simulink model "Simple_bjt"  (R2018b)
settings: Solver=FixedStepDiscrete  StartTime=0.0  StopTime=10  FixedStep=Ts  RelTol=1e-3
PreLoadFcn:
  | Ts = 1e-3
undefined symbols (not defined in the file or in its folder): DiscIntNeverNeededParam, sigbuilder_block
libraries: Simple_lib x13
settings Model: PauseTimes=455  Creator=billw  LastModifiedBy=billw
settings DataIOCC: SaveOutput=off  DSMLogging=off  SaveTime=off

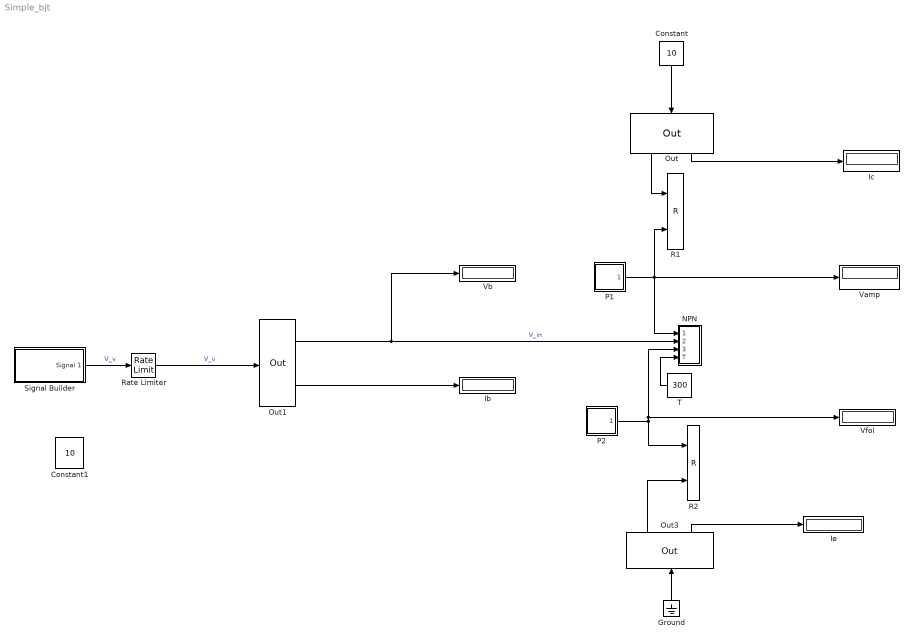
== system Simple_bjt ==
  Constant : Constant  Value=10
  Constant1 : Constant  Value=10
  Ground : Ground
  Ib : Display
  Ic : Display
  Ie : Display
  NPN : Subsystem  AncestorBlock=Simple_lib/Electronics/NPN  mask{alpha_F=0.98, alpha_R=0.9}
      mask Display:
      | patch([0 0 0.1 0.1],[-.7 1 1 -.7])
      | patch([0 0 0.1 0.1],[-1 -.7 -.7 -1],[.9 .5 .1])
      | 
      | plot([0 1],[0.25 1])
      | plot([0 1],[-0.25 -1])
      | 
      | patch([.8 1 1],[-1 -1 -0.8])
  Out : Simple_lib/Electronics/Out  Tag=Electrical
      mask init:
      | initOutput
      mask Display:
      | % This is a new mask on top of the base mask.
      | % Use "View base mask" link below to see the base mask.
      | % Icon for flow out
      | %% Complex icon
      | %plot([0 1 1], [0 0 0.4])
      | %plot([1 1 3], [0.6 1 1])
      | %plot([1 3 2 1 0 2], [0.6 0.6 0.4 0.6 0.4 0.4])
      | %patch([0 2 1],[0.4 0.4 0.6])
      | %plot([3 2 2], [1 1 0.6])
      | %plot([2.2 2.2], [1 0.6])
      | %plot([1.8 1.8], [1 0.6])
      | %plot([1.6 2.4], [0 0])
      | %plot([2 2], [0.1 -0.1])
      | %plot([2 2], [0.4 0.2])
      | %plot([2 2 3], [-0.2 -1 -1])
      | 
      | %color('white')
      | %plot([0 3], [2 2])
      | %plot([0 3], [-2 -2])
      | 
      | %% Bolder icon
      | plot([-1 0 1], [0 -1 0])
      | %patch([-1 1 0 -1], [1 1 2 1]*1-1)
      | patch([-1 -.2 -.2], [0 0 1])
      | patch([1 .2 .2], [0 0 1])
      | %patch( [-0.1 0.1 0.1 -0.1], [0 0 1 1], [1 1 1])
      | 
      | color('white')
      | plot( [-1 1], [2 2])
      | plot( [-1 1], -[2 2])
  Out1 : Simple_lib/Electronics/Out  Tag=Electrical
      mask init:
      | initOutput
      mask Display:
      | % This is a new mask on top of the base mask.
      | % Use "View base mask" link below to see the base mask.
      | % Icon for flow out
      | %% Complex icon
      | %plot([0 1 1], [0 0 0.4])
      | %plot([1 1 3], [0.6 1 1])
      | %plot([1 3 2 1 0 2], [0.6 0.6 0.4 0.6 0.4 0.4])
      | %patch([0 2 1],[0.4 0.4 0.6])
      | %plot([3 2 2], [1 1 0.6])
      | %plot([2.2 2.2], [1 0.6])
      | %plot([1.8 1.8], [1 0.6])
      | %plot([1.6 2.4], [0 0])
      | %plot([2 2], [0.1 -0.1])
      | %plot([2 2], [0.4 0.2])
      | %plot([2 2 3], [-0.2 -1 -1])
      | 
      | %color('white')
      | %plot([0 3], [2 2])
      | %plot([0 3], [-2 -2])
      | 
      | %% Bolder icon
      | plot([-1 0 1], [0 -1 0])
      | %patch([-1 1 0 -1], [1 1 2 1]*1-1)
      | patch([-1 -.2 -.2], [0 0 1])
      | patch([1 .2 .2], [0 0 1])
      | %patch( [-0.1 0.1 0.1 -0.1], [0 0 1 1], [1 1 1])
      | 
      | color('white')
      | plot( [-1 1], [2 2])
      | plot( [-1 1], -[2 2])
  Out3 : Simple_lib/Electronics/Out  Tag=Electrical
      mask init:
      | initOutput
      mask Display:
      | % This is a new mask on top of the base mask.
      | % Use "View base mask" link below to see the base mask.
      | % Icon for flow out
      | %% Complex icon
      | %plot([0 1 1], [0 0 0.4])
      | %plot([1 1 3], [0.6 1 1])
      | %plot([1 3 2 1 0 2], [0.6 0.6 0.4 0.6 0.4 0.4])
      | %patch([0 2 1],[0.4 0.4 0.6])
      | %plot([3 2 2], [1 1 0.6])
      | %plot([2.2 2.2], [1 0.6])
      | %plot([1.8 1.8], [1 0.6])
      | %plot([1.6 2.4], [0 0])
      | %plot([2 2], [0.1 -0.1])
      | %plot([2 2], [0.4 0.2])
      | %plot([2 2 3], [-0.2 -1 -1])
      | 
      | %color('white')
      | %plot([0 3], [2 2])
      | %plot([0 3], [-2 -2])
      | 
      | %% Bolder icon
      | plot([-1 0 1], [0 -1 0])
      | %patch([-1 1 0 -1], [1 1 2 1]*1-1)
      | patch([-1 -.2 -.2], [0 0 1])
      | patch([1 .2 .2], [0 0 1])
      | %patch( [-0.1 0.1 0.1 -0.1], [0 0 1 1], [1 1 1])
      | 
      | color('white')
      | plot( [-1 1], [2 2])
      | plot( [-1 1], -[2 2])
  P1 : Subsystem  AncestorBlock=Simple_lib/Electronics/P
      mask Display: disp(get(gcbh,'Name'))
  P2 : Subsystem  AncestorBlock=Simple_lib/Electronics/P
      mask Display: disp(get(gcbh,'Name'))
  R1 : Simple_lib/Electronics/R  R=5e3
      settings: AttributesFormatString=%<R> Ohms
  R2 : Simple_lib/Electronics/R  R=1e3
      settings: AttributesFormatString=%<R> Ohms
  Rate Limiter : RateLimiter  RisingSlewLimit=10  FallingSlewLimit=-10  SampleTimeMode=inherited  LinearizeAsGain=off
  Signal Builder : Subsystem  Tag=STV Subsys  LoadFcn=sigbuilder_block('load',[342 162.6 550.8 400.2 ]);  StartFcn=sigbuilder_block('start');  StopFcn=sigbuilder_block('stop');  ClipboardFcn=sigbuilder_block('clipboard');  mask(Sigbuilder block){tuvar=[0:10]}
      mask help: Simulink:masks:SigbuilderBlock_MD
      mask init:
      | if ~strcmp(get_param(bdroot(gcbh),'SimulationStatus'),'stopped') tuvar = sigbuilder_block('maskInit'); end
      settings: CopyFcn=sigbuilder_block('copy');  DeleteFcn=sigbuilder_block('delete');  ModelCloseFcn=sigbuilder_block('modelClose');  PreSaveFcn=sigbuilder_block('preSave');  PauseFcn=sigbuilder_block('pause');  ContinueFcn=sigbuilder_block('continue');  NameChangeFcn=sigbuilder_block('namechange');  OpenFcn=sigbuilder_block('open',[437.6 199.2 550.4 400 ]);  CloseFcn=sigbuilder_block('close');
      mask Display: plot(0, 0, 100, 100,[2, 2, 32, 32, 2], [68, 8, 8, 68, 68],[32, 2], [38, 38], [32, 19, 2],[53, 60, 44], [32, 17, 17, 2],[16, 16, 31, 31]);txt = getActiveGroup(gcbh);text(2, 100, txt,'verticalAlignment', 'top');
  T : Constant  Value=300
  Vamp : Display
  Vb : Display
  Vfol : Display
  wires:
  Signal Builder/1(Signal 1) -> Rate Limiter/1  "V_v"
  P1/1(Out1) -> R1/2, Vamp/1, NPN/1(Collector)
  Out/2 -> Ic/1
  Out3/1 -> R2/2
  Out1/1 -> Vb/1, NPN/2(Base)  "V_in"
  Constant/1 -> Out/1
  Out1/2 -> Ib/1
  Out/1 -> R1/1
  T/1 -> NPN/4(T)
  P2/1(Out1) -> NPN/3(Emitter), Vfol/1, R2/1
  Rate Limiter/1 -> Out1/1  "V_v"
  Ground/1 -> Out3/1
  Out3/2 -> Ie/1

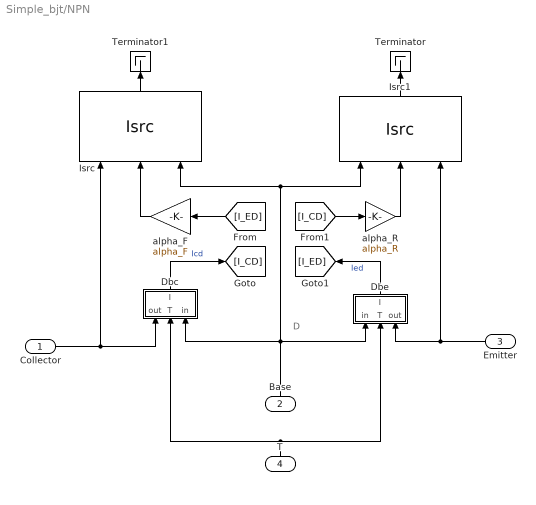
== system Simple_bjt/NPN ==
  note: D
  Collector : Inport
  Base : Inport  Port=2
  Emitter : Inport  Port=3
  T : Inport  Port=4
  Dbc : Subsystem  AncestorBlock=Simple_lib/Electronics/D  mask{I_S=1e-12}
      mask Display:
      | %plot( [ -1 0 0 ],[-1 -1 -0.3 ])
      | %plot( [ 0 0 -1],[ 0.3 1 1])
      | plot( [ -1 1],-[1 1]*1.3)
      | plot([-1 1 0 -1],[1 1 -1 1]*1.3)
      | color('white')
      | plot([-1 1], [-2 -2])
      | plot([-1 1], [2 2])
      | %port_label('input', 1, '1')
  Dbe : Subsystem  AncestorBlock=Simple_lib/Electronics/D  mask{I_S=1e-12}
      mask Display:
      | %plot( [ -1 0 0 ],[-1 -1 -0.3 ])
      | %plot( [ 0 0 -1],[ 0.3 1 1])
      | plot( [ -1 1],-[1 1]*1.3)
      | plot([-1 1 0 -1],[1 1 -1 1]*1.3)
      | color('white')
      | plot([-1 1], [-2 -2])
      | plot([-1 1], [2 2])
      | %port_label('input', 1, '1')
  Isrc : Simple_lib/Electronics/Isrc  SystemSampleTime=-1
  Isrc1 : Simple_lib/Electronics/Isrc  SystemSampleTime=-1
  Terminator : Terminator
  Terminator1 : Terminator
  alpha_F : Gain  Gain=alpha_F
  alpha_R : Gain  Gain=alpha_R
  wires:
  T/1 -> Dbc/2(T), Dbe/2(T)
  Base/1 -> Dbe/1(in), Isrc1/3, Isrc/3, Dbc/1(in)
  Dbe/1(I) -> [I_ED]  "Ied"
  alpha_R/1 -> Isrc1/2
  [I_CD] -> alpha_R/1
  alpha_F/1 -> Isrc/2
  [I_ED] -> alpha_F/1
  Dbc/1(I) -> [I_CD]  "Icd"
  Collector/1 -> Isrc/1, Dbc/3(out)
  Emitter/1 -> Dbe/3(out), Isrc1/1
  Isrc1/1 -> Terminator/1
  Isrc/1 -> Terminator1/1

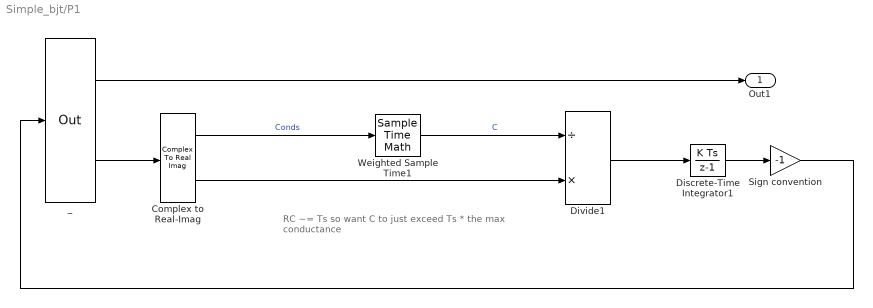
== system Simple_bjt/P1 ==
  note: RC ~= Ts
      | so want C to just exceed Ts * the max conductance
  Complex to Real-Imag : ComplexToRealImag
  Discrete-Time Integrator1 : DiscreteIntegrator  gainval=1  SampleTime=-1  LimitOutput=on  UpperSaturationLimit=1e3  LowerSaturationLimit=-1e3  ICPrevOutput=DiscIntNeverNeededParam  ICPrevScaledInput=DiscIntNeverNeededParam
  Divide1 : Product  Inputs=/*
  Sign convention : Gain  Gain=-1
  Weighted Sample Time1 : SampleTimeMath  TsampMathOp=*  weightValue=uu
  _ : Simple_lib/Electronics/Out  Tag=Electrical
      mask init:
      | initOutput
      mask Display:
      | % This is a new mask on top of the base mask.
      | % Use "View base mask" link below to see the base mask.
      | % Icon for flow out
      | %% Complex icon
      | %plot([0 1 1], [0 0 0.4])
      | %plot([1 1 3], [0.6 1 1])
      | %plot([1 3 2 1 0 2], [0.6 0.6 0.4 0.6 0.4 0.4])
      | %patch([0 2 1],[0.4 0.4 0.6])
      | %plot([3 2 2], [1 1 0.6])
      | %plot([2.2 2.2], [1 0.6])
      | %plot([1.8 1.8], [1 0.6])
      | %plot([1.6 2.4], [0 0])
      | %plot([2 2], [0.1 -0.1])
      | %plot([2 2], [0.4 0.2])
      | %plot([2 2 3], [-0.2 -1 -1])
      | 
      | %color('white')
      | %plot([0 3], [2 2])
      | %plot([0 3], [-2 -2])
      | 
      | %% Bolder icon
      | plot([-1 0 1], [0 -1 0])
      | %patch([-1 1 0 -1], [1 1 2 1]*1-1)
      | patch([-1 -.2 -.2], [0 0 1])
      | patch([1 .2 .2], [0 0 1])
      | %patch( [-0.1 0.1 0.1 -0.1], [0 0 1 1], [1 1 1])
      | 
      | color('white')
      | plot( [-1 1], [2 2])
      | plot( [-1 1], -[2 2])
  Out1 : Outport
  wires:
  Sign convention/1 -> _/1
  Complex to Real-Imag/2 -> Divide1/2
  Complex to Real-Imag/1 -> Weighted Sample Time1/1  "Conds"
  Divide1/1 -> Discrete-Time Integrator1/1
  Discrete-Time Integrator1/1 -> Sign convention/1
  _/2 -> Complex to Real-Imag/1
  _/1 -> Out1/1
  Weighted Sample Time1/1 -> Divide1/1  "C"

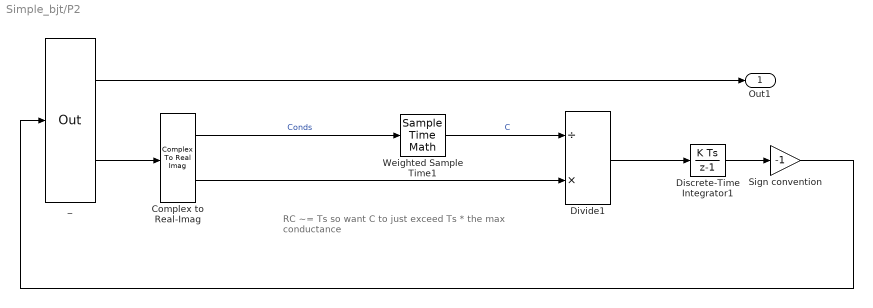
== system Simple_bjt/P2 ==
  note: RC ~= Ts
      | so want C to just exceed Ts * the max conductance
  Complex to Real-Imag : ComplexToRealImag
  Discrete-Time Integrator1 : DiscreteIntegrator  gainval=1  SampleTime=-1  LimitOutput=on  UpperSaturationLimit=1e3  LowerSaturationLimit=-1e3  ICPrevOutput=DiscIntNeverNeededParam  ICPrevScaledInput=DiscIntNeverNeededParam
  Divide1 : Product  Inputs=/*
  Sign convention : Gain  Gain=-1
  Weighted Sample Time1 : SampleTimeMath  TsampMathOp=*  weightValue=uu
  _ : Simple_lib/Electronics/Out  Tag=Electrical
      mask init:
      | initOutput
      mask Display:
      | % This is a new mask on top of the base mask.
      | % Use "View base mask" link below to see the base mask.
      | % Icon for flow out
      | %% Complex icon
      | %plot([0 1 1], [0 0 0.4])
      | %plot([1 1 3], [0.6 1 1])
      | %plot([1 3 2 1 0 2], [0.6 0.6 0.4 0.6 0.4 0.4])
      | %patch([0 2 1],[0.4 0.4 0.6])
      | %plot([3 2 2], [1 1 0.6])
      | %plot([2.2 2.2], [1 0.6])
      | %plot([1.8 1.8], [1 0.6])
      | %plot([1.6 2.4], [0 0])
      | %plot([2 2], [0.1 -0.1])
      | %plot([2 2], [0.4 0.2])
      | %plot([2 2 3], [-0.2 -1 -1])
      | 
      | %color('white')
      | %plot([0 3], [2 2])
      | %plot([0 3], [-2 -2])
      | 
      | %% Bolder icon
      | plot([-1 0 1], [0 -1 0])
      | %patch([-1 1 0 -1], [1 1 2 1]*1-1)
      | patch([-1 -.2 -.2], [0 0 1])
      | patch([1 .2 .2], [0 0 1])
      | %patch( [-0.1 0.1 0.1 -0.1], [0 0 1 1], [1 1 1])
      | 
      | color('white')
      | plot( [-1 1], [2 2])
      | plot( [-1 1], -[2 2])
  Out1 : Outport
  wires:
  Sign convention/1 -> _/1
  Complex to Real-Imag/2 -> Divide1/2
  Complex to Real-Imag/1 -> Weighted Sample Time1/1  "Conds"
  Divide1/1 -> Discrete-Time Integrator1/1
  Discrete-Time Integrator1/1 -> Sign convention/1
  _/2 -> Complex to Real-Imag/1
  _/1 -> Out1/1
  Weighted Sample Time1/1 -> Divide1/1  "C"

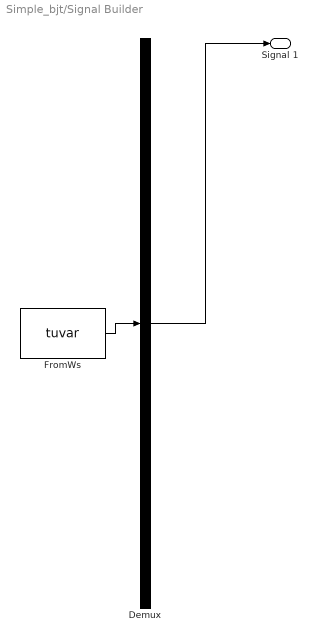
== system Simple_bjt/Signal Builder ==
  Demux : Demux  Tag=STV Demux  Outputs=1
  FromWs : FromWorkspace  Tag=STV FromWs  VariableName=tuvar  SampleTime=0
      SigBuilderData=|
      | common.afterFinalStr = 'Extrapolate'
      | common.sampleTime = 0
      | dataSet.timeRange = [0 10]
      | dataSet.name = 'Group 1'
      | sbobj.Groups.Name = 'Group 1'
      | sbobj.Groups.Signals.Name = 'Signal 1'
      | sbobj.Groups.Signals.XData = [0 0.96 0.96 2 2 4 4 6 6 7 7 7.98 7.98 10]
      | sbobj.Groups.Signals.YData = [0 0 0.3 0.3 0 0 0.395 1.44 0 0 8.75 8.75 0 0]
  Signal 1 : Outport  Tag=STV Outport
  wires:
  Demux/1 -> Signal 1/1
  FromWs/1 -> Demux/1

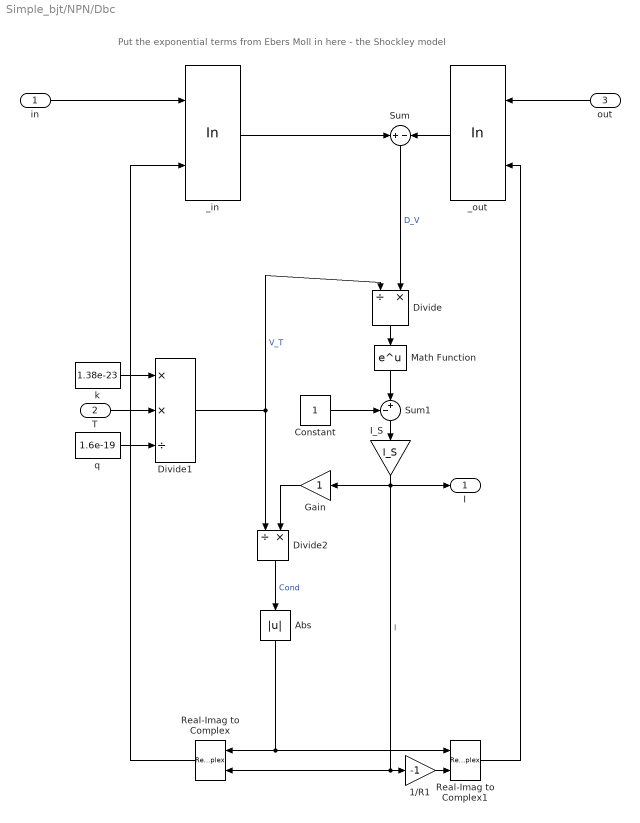
== system Simple_bjt/NPN/Dbc ==
  note: Put the exponential terms from Ebers Moll in here - the Shockley model
  in : Inport
  T : Inport  Port=2
  out : Inport  Port=3
  1/R1 : Gain  Gain=-1
  Abs : Abs
  Constant : Constant
  Divide : Product  Inputs=/*
  Divide1 : Product  Inputs=**/
  Divide2 : Product  Inputs=/*
  Gain : Gain
  I_S : Gain  Gain=I_S
  Math Function : Math  SaturateOnIntegerOverflow=on
  Real-Imag to Complex : RealImagToComplex
  Real-Imag to Complex1 : RealImagToComplex
  Sum : Sum  Inputs=+|-
  Sum1 : Sum  Inputs=-+|
  _in : Simple_lib/Electronics/In
      mask init:
      | initInput
      mask Display:
      | % This is a new mask on top of the base mask.
      | % Use "View base mask" link below to see the base mask.
      | %% Icon for flow in
      | % Signally design
      | %plot([0 2 2 3], [1 1 0 0])
      | %plot([1 3 2 1 0 2], [0.6 0.6 0.4 0.6 0.4 0.4])
      | %patch([1 3 2],[0.6 0.6 0.4])
      | %plot([0 1 1], [1 1 0.6])
      | %plot([1 1 0], [0.4 -1 -1])
      | 
      | %color('white')
      | %plot([0 3], [2 2])
      | %plot([0 3], [-2 -2])
      | 
      | %% Bolder design
      | %patch( [0 1 -1], [0 1 1])
      | patch( [-0.1 -0.1 -1], [0.95 0 0.95])
      | patch( [0.1 0.1 1], [1 0 1])
      | plot( [0.1 1 -1 -0.1], [0 -2 -2 0]*0.5)
      | %patch( [-0.1 0.1 0.1 -0.1], [0 0 1 1], [1 1 1])
      | %patch( [-1 0.1 0.1 -1], [1 1 0.95 0.95], [1 1 1])
      | 
      | %% Size the box
      | color('white')
      | plot( [-1 1], [2 2])
      | plot( [-1 1], -[2 2])
  _out : Simple_lib/Electronics/In
      mask init:
      | initInput
      mask Display:
      | % This is a new mask on top of the base mask.
      | % Use "View base mask" link below to see the base mask.
      | %% Icon for flow in
      | % Signally design
      | %plot([0 2 2 3], [1 1 0 0])
      | %plot([1 3 2 1 0 2], [0.6 0.6 0.4 0.6 0.4 0.4])
      | %patch([1 3 2],[0.6 0.6 0.4])
      | %plot([0 1 1], [1 1 0.6])
      | %plot([1 1 0], [0.4 -1 -1])
      | 
      | %color('white')
      | %plot([0 3], [2 2])
      | %plot([0 3], [-2 -2])
      | 
      | %% Bolder design
      | %patch( [0 1 -1], [0 1 1])
      | patch( [-0.1 -0.1 -1], [0.95 0 0.95])
      | patch( [0.1 0.1 1], [1 0 1])
      | plot( [0.1 1 -1 -0.1], [0 -2 -2 0]*0.5)
      | %patch( [-0.1 0.1 0.1 -0.1], [0 0 1 1], [1 1 1])
      | %patch( [-1 0.1 0.1 -1], [1 1 0.95 0.95], [1 1 1])
      | 
      | %% Size the box
      | color('white')
      | plot( [-1 1], [2 2])
      | plot( [-1 1], -[2 2])
  k : Constant  Value=1.38e-23
  q : Constant  Value=1.6e-19
  I : Outport
  wires:
  Real-Imag to Complex1/1 -> _out/2
  Divide2/1 -> Abs/1  "Cond"
  I_S/1 -> Real-Imag to Complex/2, 1/R1/1, Gain/1, I/1  "I"
  _out/1 -> Sum/2
  Math Function/1 -> Sum1/2
  Constant/1 -> Sum1/1
  Sum1/1 -> I_S/1
  out/1 -> _out/1
  Sum/1 -> Divide/2  "D_V"
  _in/1 -> Sum/1
  in/1 -> _in/1
  Divide/1 -> Math Function/1
  T/1 -> Divide1/2
  q/1 -> Divide1/3
  Divide1/1 -> Divide2/1, Divide/1  "V_T"
  k/1 -> Divide1/1
  Gain/1 -> Divide2/2
  Abs/1 -> Real-Imag to Complex1/1, Real-Imag to Complex/1
  Real-Imag to Complex/1 -> _in/2
  1/R1/1 -> Real-Imag to Complex1/2

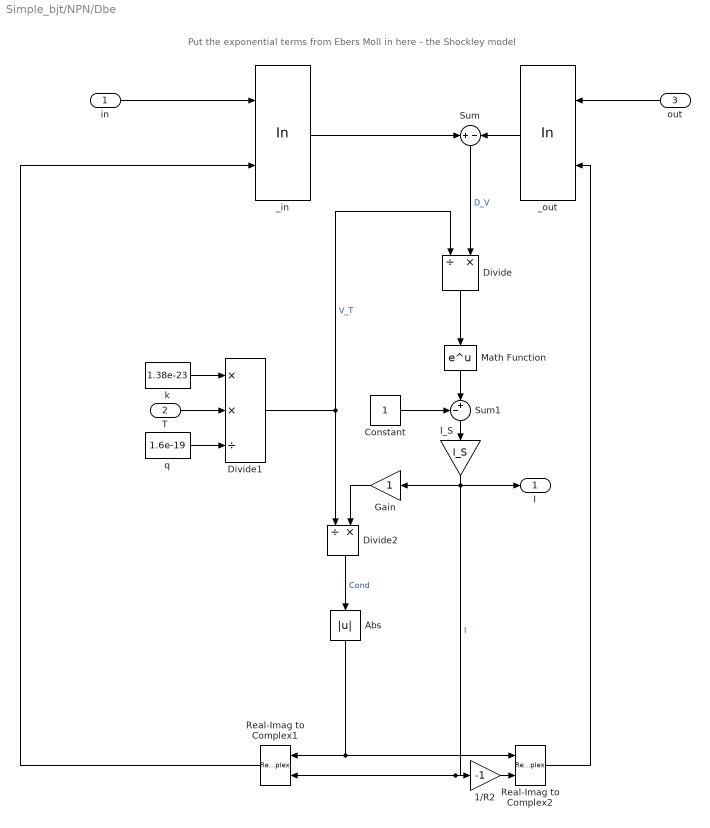
== system Simple_bjt/NPN/Dbe ==
  note: Put the exponential terms from Ebers Moll in here - the Shockley model
  in : Inport
  T : Inport  Port=2
  out : Inport  Port=3
  1/R2 : Gain  Gain=-1
  Abs : Abs
  Constant : Constant
  Divide : Product  Inputs=/*
  Divide1 : Product  Inputs=**/
  Divide2 : Product  Inputs=/*
  Gain : Gain
  I_S : Gain  Gain=I_S
  Math Function : Math  SaturateOnIntegerOverflow=on
  Real-Imag to Complex1 : RealImagToComplex
  Real-Imag to Complex2 : RealImagToComplex
  Sum : Sum  Inputs=+|-
  Sum1 : Sum  Inputs=-+|
  _in : Simple_lib/Electronics/In
      mask init:
      | initInput
      mask Display:
      | % This is a new mask on top of the base mask.
      | % Use "View base mask" link below to see the base mask.
      | %% Icon for flow in
      | % Signally design
      | %plot([0 2 2 3], [1 1 0 0])
      | %plot([1 3 2 1 0 2], [0.6 0.6 0.4 0.6 0.4 0.4])
      | %patch([1 3 2],[0.6 0.6 0.4])
      | %plot([0 1 1], [1 1 0.6])
      | %plot([1 1 0], [0.4 -1 -1])
      | 
      | %color('white')
      | %plot([0 3], [2 2])
      | %plot([0 3], [-2 -2])
      | 
      | %% Bolder design
      | %patch( [0 1 -1], [0 1 1])
      | patch( [-0.1 -0.1 -1], [0.95 0 0.95])
      | patch( [0.1 0.1 1], [1 0 1])
      | plot( [0.1 1 -1 -0.1], [0 -2 -2 0]*0.5)
      | %patch( [-0.1 0.1 0.1 -0.1], [0 0 1 1], [1 1 1])
      | %patch( [-1 0.1 0.1 -1], [1 1 0.95 0.95], [1 1 1])
      | 
      | %% Size the box
      | color('white')
      | plot( [-1 1], [2 2])
      | plot( [-1 1], -[2 2])
  _out : Simple_lib/Electronics/In
      mask init:
      | initInput
      mask Display:
      | % This is a new mask on top of the base mask.
      | % Use "View base mask" link below to see the base mask.
      | %% Icon for flow in
      | % Signally design
      | %plot([0 2 2 3], [1 1 0 0])
      | %plot([1 3 2 1 0 2], [0.6 0.6 0.4 0.6 0.4 0.4])
      | %patch([1 3 2],[0.6 0.6 0.4])
      | %plot([0 1 1], [1 1 0.6])
      | %plot([1 1 0], [0.4 -1 -1])
      | 
      | %color('white')
      | %plot([0 3], [2 2])
      | %plot([0 3], [-2 -2])
      | 
      | %% Bolder design
      | %patch( [0 1 -1], [0 1 1])
      | patch( [-0.1 -0.1 -1], [0.95 0 0.95])
      | patch( [0.1 0.1 1], [1 0 1])
      | plot( [0.1 1 -1 -0.1], [0 -2 -2 0]*0.5)
      | %patch( [-0.1 0.1 0.1 -0.1], [0 0 1 1], [1 1 1])
      | %patch( [-1 0.1 0.1 -1], [1 1 0.95 0.95], [1 1 1])
      | 
      | %% Size the box
      | color('white')
      | plot( [-1 1], [2 2])
      | plot( [-1 1], -[2 2])
  k : Constant  Value=1.38e-23
  q : Constant  Value=1.6e-19
  I : Outport
  wires:
  Real-Imag to Complex2/1 -> _out/2
  Divide2/1 -> Abs/1  "Cond"
  I_S/1 -> Real-Imag to Complex1/2, 1/R2/1, Gain/1, I/1  "I"
  _out/1 -> Sum/2
  Math Function/1 -> Sum1/2
  Constant/1 -> Sum1/1
  Sum1/1 -> I_S/1
  out/1 -> _out/1
  Sum/1 -> Divide/2  "D_V"
  _in/1 -> Sum/1
  in/1 -> _in/1
  Divide/1 -> Math Function/1
  T/1 -> Divide1/2
  q/1 -> Divide1/3
  Divide1/1 -> Divide2/1, Divide/1  "V_T"
  k/1 -> Divide1/1
  Gain/1 -> Divide2/2
  Abs/1 -> Real-Imag to Complex1/1, Real-Imag to Complex2/1
  1/R2/1 -> Real-Imag to Complex2/2
  Real-Imag to Complex1/1 -> _in/2
